simulink model "mcb_pmsm_foc_hall_dsPIC33CK256MP508"  (R2022a)
settings: Solver=FixedStepDiscrete  StartTime=0.0  StopTime=10.0  FixedStep=50e-6  RelTol=1e-3  EnableMultiTasking=on
PreLoadFcn:
  | mcb_pmsm_foc_hall_lvmc_data;
InitFcn:
  | mcb_pmsm_foc_hall_lvmc_data;
undefined symbols (not defined in the file or in its folder): A0, AN0, B0, D13, MaxPer, ms, P32, P77, Pin, pmsm, PWM1max, Resol, s, us
libraries: MCHP_Blockset x19, simulink x3
(part 2 of 2)

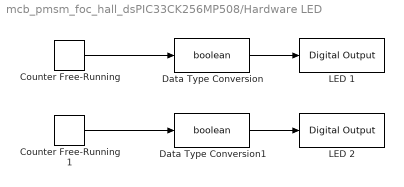
== system mcb_pmsm_foc_hall_dsPIC33CK256MP508/Hardware LED ==
  Counter Free-Running : simulink/Sources/Counter Free-Running  NumBits=1  tsamp=0.5
  Counter Free-Running1 : simulink/Sources/Counter Free-Running  NumBits=1  tsamp=0.1
  Data Type Conversion : DataTypeConversion  OutDataTypeStr=boolean  SaturateOnIntegerOverflow=off  RndMeth=Floor
  Data Type Conversion1 : DataTypeConversion  OutDataTypeStr=boolean  SaturateOnIntegerOverflow=off  RndMeth=Floor
  LED 1 : MCHP_Blockset/Digital IO/Digital Output  PORT=Dynamic Options  PORT_TXT="E   [ 0 : 15 ]"  PIN=6  PACK=off  SIMULTANEOUS=off  READPREVIOUS=off  ORDERING=None  SampleTime=-1  MCHP_MASTERLINK=mcb_pmsm_foc_hall_dsPIC33CK256MP508/Hardware Init/Microchip Master
      settings: SourceProductName=MPLAB Device Blocks for Simulink
  LED 2 : MCHP_Blockset/Digital IO/Digital Output  PORT=Dynamic Options  PORT_TXT="E   [ 0 : 15 ]"  PIN=7  PACK=off  SIMULTANEOUS=off  READPREVIOUS=off  ORDERING=None  SampleTime=-1  MCHP_MASTERLINK=mcb_pmsm_foc_hall_dsPIC33CK256MP508/Hardware Init/Microchip Master
      settings: SourceProductName=MPLAB Device Blocks for Simulink
  wires:
  Counter Free-Running1/1 -> Data Type Conversion1/1
  Data Type Conversion/1 -> LED 1/1
  Counter Free-Running/1 -> Data Type Conversion/1
  Data Type Conversion1/1 -> LED 2/1

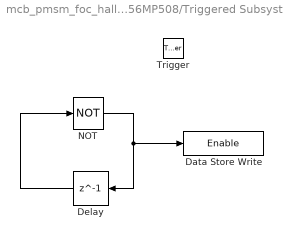
== system mcb_pmsm_foc_hall_dsPIC33CK256MP508/Triggered Subsystem ==
  Trigger : TriggerPort  TriggerType=falling  VariantControl=Variant
  Data Store Write : DataStoreWrite  DataStoreName=Enable  IndexOptions=Index vector (dialog)  Indices=1  OutputSizes=1
  Delay : Delay  DelayLength=1  InitialCondition=0
  NOT : Logic  Operator=NOT  IconShape=distinctive  AllPortsSameDT=off  OutDataTypeStr=boolean
  wires:
  Delay/1 -> NOT/1
  NOT/1 -> Delay/1, Data Store Write/1

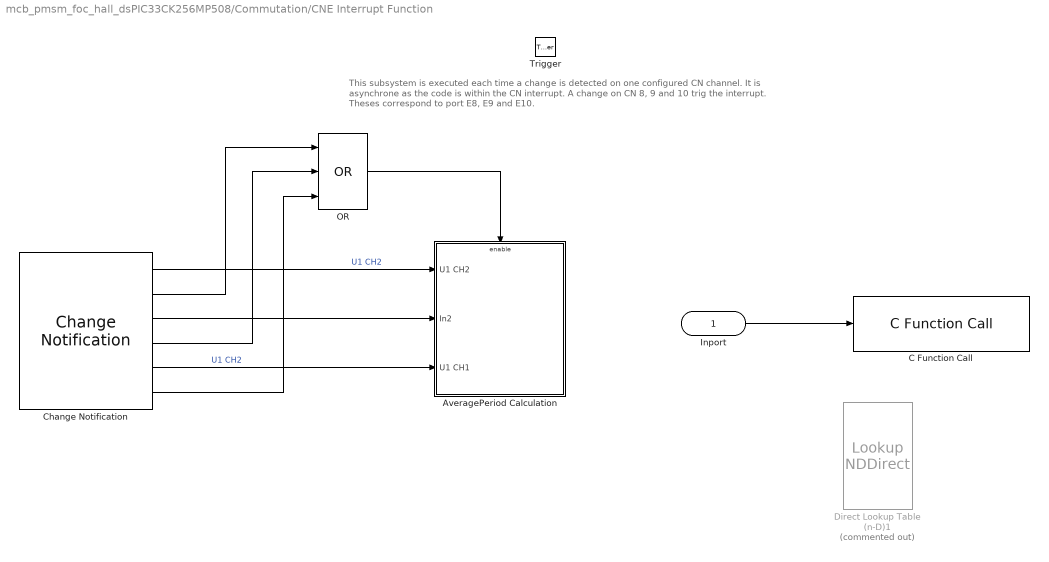
== system mcb_pmsm_foc_hall_dsPIC33CK256MP508/Commutation/CNE Interrupt Function ==
  note: This subsystem is executed each time a change is detected on one configured CN channel.
      | It is asynchrone as the code is within the CN interrupt.
      | A change on CN 8, 9 and 10 trig the interrupt. Theses correspond to port E8, E9 and E10.
  Inport : Inport
  Trigger : TriggerPort  TriggerType=function-call  VariantControl=(inherit)  PortDimensions=1
  AveragePeriod Calculation : Subsystem
  C Function Call : MCHP_Blockset/User Functions/C Function Call  ParseFilesChkbx=on  ListFunctions1=Custom Function  Function1=void myPWMOverrideEnable(unsigned int sector)  AddHeaderDeclaration=on  Function1Type=when block is updated (default)  Fct1BlockIn=sector  FctReturnBlockOut=on  DataCollected="s.chksm={ '51328-Jul-2022 14:38:31'};s.File1={ '  void  myPWMOverrideEnable(unsigned int sector)'};"  ORDERING=None  SampleTime=-1  S_INPUT=0  S_INPUT_Size=0  S_OUTPUT=0  S_OUTPUT_Size=0  S_ListCustomDatatype=0  MCHP_CRC=1083330  MCHP_MASTERLINK=mcb_pmsm_foc_hall_dsPIC33CK256MP508/Hardware Init/Microchip Master  PinDigitalInput=[]  PinDigitalOutput=[]  PinAnalogInput=[]
      settings: SourceProductName=MPLAB Device Blocks for Simulink
  Change Notification : MCHP_Blockset/Pulse Input//Output/Change Notification  IntPriority=7  Channel="[19    20    21]"  Channel_EP="[  E8  E9  E10]"  Channel_OLD="[72  73  74]"  Channel_UP_Down_Periode="[4     4     4]"  MaxChannel="[0.0419424   0.0419424   0.0419424]"  SafeMarge="[0     0     0]"  MaxChannelValue="2.^[ 16.000  16.000  16.000]  =>  [65534  65534  65534]"  CNxmax="[65534  65534  65534]"  Timer="[1  1  1]"  ChangeDetected="[1     1     1]"  OutputPortValue="[0     0     0]"  evalin_ws=CNE8max=MCHP_Fun.Hex2num('40EFFFC000000000');CNE9max=MCHP_Fun.Hex2num('40EFFFC000000000');CNE10max=MCHP_Fun.Hex2num('40EFFFC000000000');  SampleTime=-1  Status=OK  MCHP_PORT={Change Notification E8}{CNE8}9:0:E8;{Change Notification E9}{CNE9}9:0:E9;{Change Notification E10}{CNE10}9:0:E10;  MCHP_TIMER_REQUEST={Change Notification 72}{CNE8}7:1:1:0:[]:4194240;{Change Notification 73}{CNE9}7:1:1:0:[]:4194240;{Change Notification 74}{CNE10}7:1:1:0:[]:4194240;  MCHP_TIMER_RESULT=[1 65534.00000000007276 ;1 65534.00000000007276 ;1 65534.00000000007276 ]  MCHP_USER_INTERRUPTS={CNEIE}{CNE}{Change Notification - E}{7};  MCHP_MASTERLINK=mcb_pmsm_foc_hall_dsPIC33CK256MP508/Hardware Init/Microchip Master
      settings: SourceProductName=MPLAB Device Blocks for Simulink
  Direct Lookup Table (n-D)1 : LookupNDDirect  Commented=on  NumberOfTableDimensions=1  Table=[0 0 5460 2730 10920 13650 8190 0]  TableDataTypeStr=uint16
  OR : Logic  Operator=OR  Inputs=3  IconShape=distinctive  AllPortsSameDT=off  OutDataTypeStr=boolean
  wires:
  OR/1 -> AveragePeriod Calculation/Enable
  Change Notification/5 -> AveragePeriod Calculation/3(U1 CH1)  "U1 CH2"
  Change Notification/3 -> AveragePeriod Calculation/2(In2)
  Change Notification/1 -> AveragePeriod Calculation/1(U1 CH2)  "U1 CH2"
  Change Notification/6 -> OR/3
  Change Notification/4 -> OR/2
  Change Notification/2 -> OR/1
  Inport/1 -> C Function Call/1

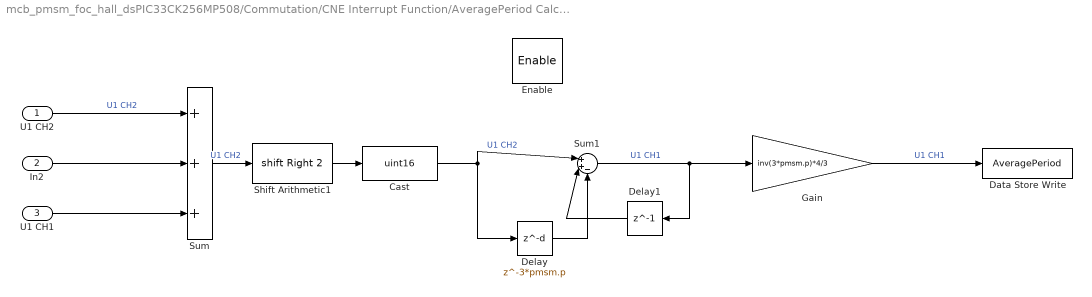
== system mcb_pmsm_foc_hall_dsPIC33CK256MP508/Commutation/CNE Interrupt Function/AveragePeriod Calculation ==
  U1 CH2 : Inport
  In2 : Inport  Port=2
  U1 CH1 : Inport  Port=3
  Enable : EnablePort
  Cast : DataTypeConversion  OutDataTypeStr=uint16  SaturateOnIntegerOverflow=off  RndMeth=Floor
  Data Store Write : DataStoreWrite  DataStoreName=AveragePeriod  IndexOptions=Index vector (dialog)  Indices=1  OutputSizes=1
  Delay : Delay  DelayLength=3*pmsm.p  InitialCondition=0  UseCircularBuffer=on
  Delay1 : Delay  DelayLength=1  InitialCondition=0
  Gain : Gain  Gain=inv(3*pmsm.p)*4/3  OutDataTypeStr=uint16
  Shift Arithmetic1 : ArithShift  BitShiftNumber=2  BitShiftDirection=Right
  Sum : Sum  Inputs=+++  AccumDataTypeStr=uint32  OutDataTypeStr=uint32
  Sum1 : Sum  Inputs=|++-  AccumDataTypeStr=int32  OutDataTypeStr=int32
  wires:
  Gain/1 -> Data Store Write/1  "U1 CH1"
  U1 CH1/1 -> Sum/3
  Delay1/1 -> Sum1/2
  Delay/1 -> Sum1/3
  Sum/1 -> Shift Arithmetic1/1  "U1 CH2"
  In2/1 -> Sum/2
  Cast/1 -> Delay/1, Sum1/1  "U1 CH2"
  Shift Arithmetic1/1 -> Cast/1
  Sum1/1 -> Gain/1, Delay1/1  "U1 CH1"
  U1 CH2/1 -> Sum/1  "U1 CH2"
